simulink model "example1_sim"  (R2018a)
settings: Solver=VariableStepAuto  StartTime=0.0  StopTime=30  RelTol=1e-3
values from neighbouring files (symbols this model uses):
  Kp = 0.6*Kcr    (= 18)    [example1.m]
  Td = 0.125*Pcr    [example1.m]
  Ti = 0.5*Pcr    [example1.m]
libraries: simulink x4
settings Model: Creator=gbecerra  LastModifiedBy=gbecerra

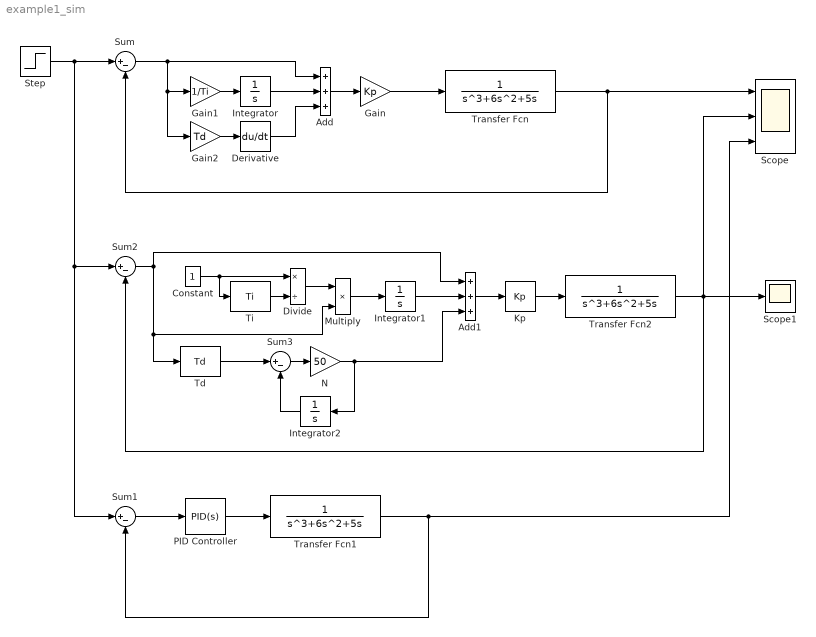
== system example1_sim ==
  Add : Sum  Inputs=+++
  Add1 : Sum  Inputs=+++
  Constant : Constant
  Derivative : Derivative
  Divide : Product  Inputs=*/
  Gain : Gain  Gain=Kp
  Gain1 : Gain  Gain=1/Ti
  Gain2 : Gain  Gain=Td
  Integrator : Integrator
  Integrator1 : Integrator
  Integrator2 : Integrator
  Kp : simulink/Math Operations/Slider Gain  gain=Kp  low=0  high=50
  Multiply : Product
  N : Gain  Gain=50
  PID Controller : simulink/Continuous/PID Controller  Controller=PID  TimeDomain=Continuous-time  SampleTime=-1  IntegratorMethod=Forward Euler  FilterMethod=Forward Euler  Form=Ideal  UseFilter=on  ControllerParametersSource=internal  P=Kp  I=1/Ti  D=Td  N=100  InitialConditionSource=internal  InitialConditionForIntegrator=0  InitialConditionForFilter=0  ExternalReset=none  LimitOutput=off  UpperSaturationLimit=inf  LowerSaturationLimit=-inf  LinearizeAsGain=on  AntiWindupMode=none  Kb=1  TrackingMode=off  Kt=1  PParamMin=[]  PParamMax=[]  IParamMin=[]  IParamMax=[]  DParamMin=[]  DParamMax=[]  NParamMin=[]  NParamMax=[]  KbParamMin=[]  KbParamMax=[]  KtParamMin=[]  KtParamMax=[]  POutMin=[]  POutMax=[]  IOutMin=[]  IOutMax=[]  DOutMin=[]  DOutMax=[]  NOutMin=[]  NOutMax=[]  KbOutMin=[]  KbOutMax=[]  KtOutMin=[]  KtOutMax=[]  IntegratorOutMin=[]  IntegratorOutMax=[]  FilterOutMin=[]  FilterOutMax=[]  SumOutMin=[]  SumOutMax=[]  SumI1OutMin=[]  SumI1OutMax=[]  SumI2OutMin=[]  SumI2OutMax=[]  SumI3OutMin=[]  SumI3OutMax=[]  SumDOutMin=[]  SumDOutMax=[]  SaturationOutMin=[]  SaturationOutMax=[]  IntegratorContinuousStateAttributes=''  IntegratorStateMustResolveToSignalObject=off  IntegratorRTWStateStorageClass=Auto  FilterContinuousStateAttributes=''  FilterStateMustResolveToSignalObject=off  FilterRTWStateStorageClass=Auto  DifferentiatorICPrevScaledInput=0  DifferentiatorOutMin=[]  DifferentiatorOutMax=[]  FilterDiffOutCoefMin=[]  FilterDiffOutCoefMax=[]  SumDenOutMin=[]  SumDenOutMax=[]  SumNumOutMin=[]  SumNumOutMax=[]  ReciprocalOutMin=[]  ReciprocalOutMax=[]  DivideOutMin=[]  DivideOutMax=[]  TunerSelectOption=Transfer Function Based (PID Tuner App)
  Scope : Scope  NumInputPorts=3
  Scope1 : Scope
  Step : Step  Time=0  SampleTime=0
  Sum{,1..3} (4 alike) : Sum  Inputs=|+-
  Td : simulink/Math Operations/Slider Gain  gain=Td  low=0  high=1
  Ti : simulink/Math Operations/Slider Gain  gain=Ti  low=0  high=4
  Transfer Fcn : TransferFcn  Denominator=[1 6 5 0]
  Transfer Fcn1 : TransferFcn  Denominator=[1 6 5 0]
  Transfer Fcn2 : TransferFcn  Denominator=[1 6 5 0]
  wires:
  Gain/1 -> Transfer Fcn/1
  Transfer Fcn/1 -> Sum/2, Scope/1
  Add/1 -> Gain/1
  Sum/1 -> Gain2/1, Gain1/1, Add/1
  Gain1/1 -> Integrator/1
  Integrator/1 -> Add/2
  Gain2/1 -> Derivative/1
  Derivative/1 -> Add/3
  Transfer Fcn1/1 -> Sum1/2, Scope/3
  PID Controller/1 -> Transfer Fcn1/1
  Sum1/1 -> PID Controller/1
  Step/1 -> Sum1/1, Sum2/1, Sum/1
  Add1/1 -> Kp/1
  Transfer Fcn2/1 -> Scope1/1, Scope/2, Sum2/2
  Kp/1 -> Transfer Fcn2/1
  Td/1 -> Sum3/1
  Sum3/1 -> N/1
  Integrator2/1 -> Sum3/2
  N/1 -> Add1/3, Integrator2/1
  Ti/1 -> Divide/2
  Constant/1 -> Ti/1, Divide/1
  Divide/1 -> Multiply/1
  Sum2/1 -> Multiply/2, Td/1, Add1/1
  Multiply/1 -> Integrator1/1
  Integrator1/1 -> Add1/2
